simulink model "System_TP"  (R2016b)
settings: Solver=VariableStepAuto  StartTime=0.0  StopTime=10.0  RelTol=1e-3
settings Model: Creator=akshita_jain  LastModifiedBy=akshita_jain

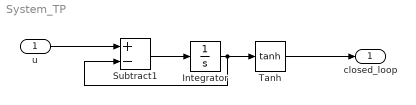
== system System_TP ==
  u : Inport
  Integrator : Integrator
  Subtract1 : Sum  Inputs=+-
  Tanh : Trigonometry  Operator=tanh
  closed_loop : Outport
  wires:
  Subtract1/1 -> Integrator/1
  Integrator/1 -> Subtract1/2, Tanh/1
  Tanh/1 -> closed_loop/1
  u/1 -> Subtract1/1
